simulink model "sum_collapse_int_test"  (Simulink 7.2)
settings: Solver=VariableStepDiscrete  StartTime=0.0  StopTime=10.0  RelTol=1e-3
settings Model: Creator=arnaud  LastModifiedBy=arnaud
settings DataIOCC: SaveFormat=Structure

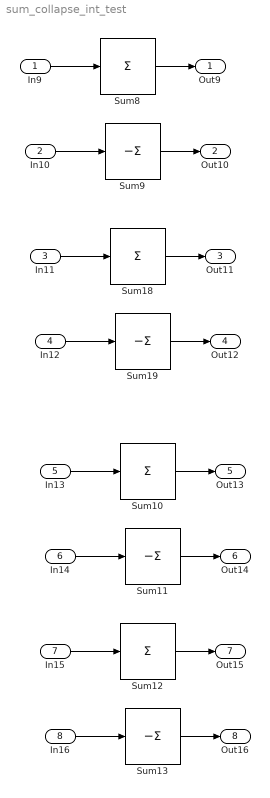
== system sum_collapse_int_test ==
  In9 : Inport  DataType=int8  OutDataType=sfix(16)  OutScaling=2^0  OutDataTypeStr=int8
  In10 : Inport  Port=2  DataType=int8  OutDataType=sfix(16)  OutScaling=2^0  OutDataTypeStr=int8
  In11 : Inport  Port=3  PortDimensions=3  DataType=int8  OutDataType=sfix(16)  OutScaling=2^0  OutDataTypeStr=int8
  In12 : Inport  Port=4  PortDimensions=3  DataType=int8  OutDataType=sfix(16)  OutScaling=2^0  OutDataTypeStr=int8
  In13 : Inport  Port=5  PortDimensions=[2 3]  DataType=int8  OutDataType=sfix(16)  OutScaling=2^0  OutDataTypeStr=int8
  In14 : Inport  Port=6  PortDimensions=[2 3]  DataType=int8  OutDataType=sfix(16)  OutScaling=2^0  OutDataTypeStr=int8
  In15 : Inport  Port=7  PortDimensions=[2 3]  DataType=int8  OutDataType=sfix(16)  OutScaling=2^0  OutDataTypeStr=int8
  In16 : Inport  Port=8  PortDimensions=[2 3]  DataType=int8  OutDataType=sfix(16)  OutScaling=2^0  OutDataTypeStr=int8
  Sum10 : Sum  Inputs=+  CollapseMode=Specified dimension  OutDataType=sfix(16)  OutScaling=2^0
  Sum11 : Sum  Inputs=-  CollapseMode=Specified dimension  OutDataType=sfix(16)  OutScaling=2^0
  Sum12 : Sum  Inputs=+  CollapseMode=Specified dimension  CollapseDim=2  OutDataType=sfix(16)  OutScaling=2^0
  Sum13 : Sum  Inputs=-  CollapseMode=Specified dimension  CollapseDim=2  OutDataType=sfix(16)  OutScaling=2^0
  Sum18 : Sum  Inputs=+  CollapseMode=Specified dimension  OutDataType=sfix(16)  OutScaling=2^0
  Sum19 : Sum  Inputs=-  CollapseMode=Specified dimension  OutDataType=sfix(16)  OutScaling=2^0
  Sum8 : Sum  Inputs=+  CollapseMode=Specified dimension  OutDataType=sfix(16)  OutScaling=2^0
  Sum9 : Sum  Inputs=-  CollapseMode=Specified dimension  OutDataType=sfix(16)  OutScaling=2^0
  Out9 : Outport  OutDataType=sfix(16)  OutScaling=2^0
  Out10 : Outport  Port=2  OutDataType=sfix(16)  OutScaling=2^0
  Out11 : Outport  Port=3  OutDataType=sfix(16)  OutScaling=2^0
  Out12 : Outport  Port=4  OutDataType=sfix(16)  OutScaling=2^0
  Out13 : Outport  Port=5  OutDataType=sfix(16)  OutScaling=2^0
  Out14 : Outport  Port=6  OutDataType=sfix(16)  OutScaling=2^0
  Out15 : Outport  Port=7  OutDataType=sfix(16)  OutScaling=2^0
  Out16 : Outport  Port=8  OutDataType=sfix(16)  OutScaling=2^0
  wires:
  In9/1 -> Sum8/1
  Sum8/1 -> Out9/1
  In10/1 -> Sum9/1
  Sum9/1 -> Out10/1
  In11/1 -> Sum18/1
  Sum18/1 -> Out11/1
  In12/1 -> Sum19/1
  Sum19/1 -> Out12/1
  In13/1 -> Sum10/1
  Sum10/1 -> Out13/1
  In14/1 -> Sum11/1
  Sum11/1 -> Out14/1
  In15/1 -> Sum12/1
  Sum12/1 -> Out15/1
  In16/1 -> Sum13/1
  Sum13/1 -> Out16/1
